simulink model "untitled"  (R2017a)
settings: Solver=FixedStepAuto  StartTime=0.0  StopTime=0.3  FixedStep=0.001  RelTol=1e-3
libraries: cstblocks x3
settings Model: Creator=Chaohua Zhao  LastModifiedBy=Chaohua Zhao

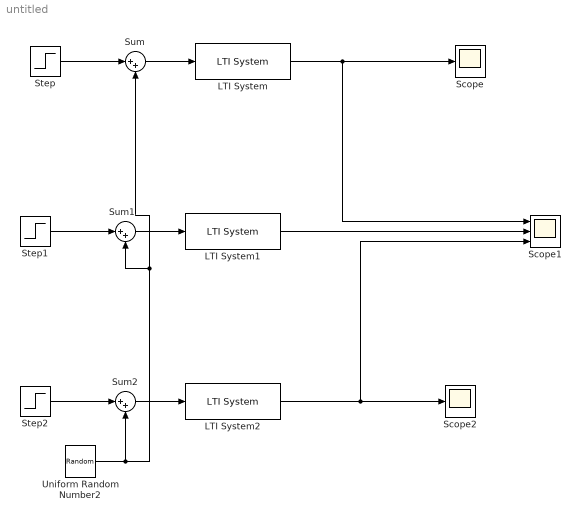
== system untitled ==
  LTI System : cstblocks/LTI System  sys=tfp  IC=[]
  LTI System1 : cstblocks/LTI System  sys=tfr  IC=[]
  LTI System2 : cstblocks/LTI System  sys=tfy  IC=[]
  Scope : Scope
  Scope1 : Scope  NumInputPorts=3
  Scope2 : Scope
  Step : Step  Time=0  SampleTime=0
  Step1 : Step  Time=0  SampleTime=0
  Step2 : Step  Time=0  SampleTime=0
  Sum : Sum  Inputs=|++
  Sum1 : Sum  Inputs=|++
  Sum2 : Sum  Inputs=|++
  Uniform Random Number2 : UniformRandomNumber  Minimum=-0.05  Maximum=0.05  SampleTime=0.001
  wires:
  LTI System/1 -> Scope1/1, Scope/1
  Uniform Random Number2/1 -> Sum2/2, Sum1/2, Sum/2
  Sum/1 -> LTI System/1
  Step/1 -> Sum/1
  Step1/1 -> Sum1/1
  Sum1/1 -> LTI System1/1
  LTI System2/1 -> Scope1/3, Scope2/1
  Sum2/1 -> LTI System2/1
  Step2/1 -> Sum2/1
  LTI System1/1 -> Scope1/2
